simulink model "Model_4"  (R2021b)
settings: Solver=VariableStepAuto  StartTime=0.0  StopTime=10.0  RelTol=1e-3
InitFcn:
  | x_ref = 1; l_ref =0.2; l_ini = 0.7;
  | 
  | %ADRC' s parameter caculation
  | b0 = (ml+mc)/(mc*ml +mc*mt+ml*mt);k_ESO = 15;T_set  = 3;
  | 
  | s_cl = -5.85/T_set;
  | Kp   = s_cl^2;
  | Kd   = -2*s_cl;
  | 
  | s_ESO = k_ESO*s_cl;
  | l1        = -3*s_ESO;
  | l2        = 3*( s_ESO)^2;
  | l3        = -(s_ESO)^3;
  | 
  | %Observer
  | A = [-l1, 1, 0;
  |         -l2, 0, 1;
  |         -l3, 0, 0];
  | B = [0;
  |         b0;
  |         0];
  | L = [l1;
  |        l2;
  |        l3];
  | 
  | b1 = (mt+mc)/(mc*ml +mc*mt+ml*mt);k_ESO1 =90;T_set1  =3;
  | s_cl1 = -5.85/T_set1;
  | Kp1   = s_cl1^2;
  | Kd1   = -2*s_cl1;
  | 
  | s_ESO1 = k_ESO1*s_cl1;
  | l11        = -3*s_ESO1;
  | l21        = 3*( s_ESO1)^2;
  | l31        = -(s_ESO1)^3;
  | 
  | %Observer
  | A1 = [-l11, 1, 0;
  |         -l21, 0, 1;
  |         -l31, 0, 0];
  | B1 = [0;
  |         b1;
  |         0];
  | L1 = [l11;
  |        l21;
  |        l31];
values from neighbouring files (symbols this model uses):
  g = 9.81    [Thong_so_double_pendulum.m]
undefined symbols (not defined in the file or in its folder): data_model41, i, l, mc, o, particle, sigbuilder_block
libraries: neural x166, simulink x5, simulink_extras x5
(part 1 of 4)
settings Model: Creator=Dao Hieu  LastModifiedBy=Admin

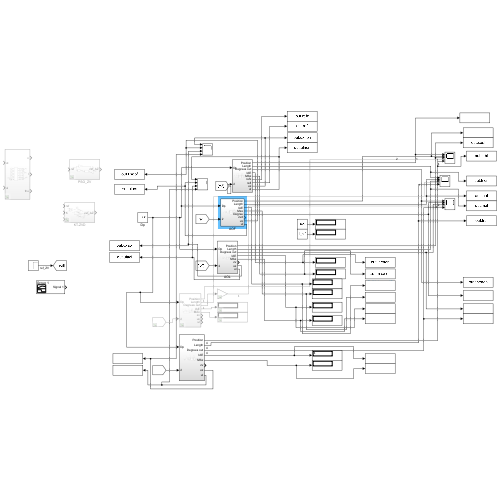
[thumbnail: Simulink's stored preview of the top-level diagram]
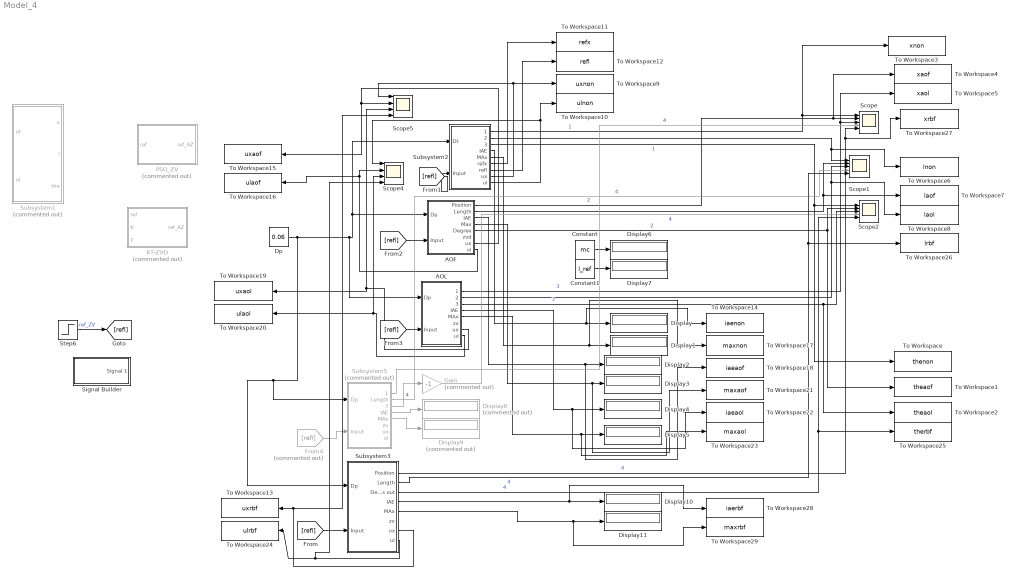
== system Model_4 ==
  AOF : Subsystem
  AOL : Subsystem
  Constant : Constant  Value=mc
  Constant1 : Constant  Value=l_ref
  Display{,1..7,10..11} (10 alike) : Display
  Display8 : Display  Commented=on
  Display9 : Display  Commented=on
  Dp : Constant  Value=0.06
  From4 : From  Commented=on  GotoTag=refl
  Gain : Gain  Commented=on  Gain=-1
  KT-ZVD : Subsystem  Commented=on
  PSO_ZV : Subsystem  Commented=on
  Scope : Scope  NumInputPorts=5
  Scope1 : Scope  NumInputPorts=5
  Scope2 : Scope  NumInputPorts=5
  Scope4 : Scope  NumInputPorts=4
  Scope5 : Scope  NumInputPorts=4
  Signal Builder : Subsystem  Tag=STV Subsys  LoadFcn=sigbuilder_block('load');  StartFcn=sigbuilder_block('start');  StopFcn=sigbuilder_block('stop');  ClipboardFcn=sigbuilder_block('clipboard');  mask(Sigbuilder block){tuvar=[0:10]}
      mask help: Simulink:masks:SigbuilderBlock_MD
      mask init:
      | if ~strcmp(get_param(bdroot(gcbh),'SimulationStatus'),'stopped') tuvar = sigbuilder_block('maskInit'); end
      settings: CopyFcn=sigbuilder_block('copy');  DeleteFcn=sigbuilder_block('delete');  ModelCloseFcn=sigbuilder_block('modelClose');  PreSaveFcn=sigbuilder_block('preSave');  PauseFcn=sigbuilder_block('pause');  ContinueFcn=sigbuilder_block('continue');  NameChangeFcn=sigbuilder_block('namechange');  OpenFcn=sigbuilder_block('open',[388.2 157.8 550.8 400.2 ]);  CloseFcn=sigbuilder_block('close');
      mask Display: plot(0, 0, 100, 100,[2, 2, 32, 32, 2], [68, 8, 8, 68, 68],[32, 2], [38, 38], [32, 19, 2],[53, 60, 44], [32, 17, 17, 2],[16, 16, 31, 31]);txt = getActiveGroup(gcbh);text(2, 100, txt,'verticalAlignment', 'top');
  Step6 : Step  Before=l_ini  After=l_ref  SampleTime=0
  Subsystem1 : Subsystem  Commented=on
  Subsystem2 : Subsystem
  Subsystem3 : Subsystem
  Subsystem5 : Subsystem  Commented=on
  To Workspace : ToWorkspace  VariableName=thenon  SampleTime=0.001
  To Workspace1 : ToWorkspace  VariableName=theaof  SampleTime=0.001
  To Workspace10 : ToWorkspace  VariableName=ulnon  SampleTime=0.001
  To Workspace11 : ToWorkspace  VariableName=refx  SampleTime=0.001
  To Workspace12 : ToWorkspace  VariableName=refl  SampleTime=0.001
  To Workspace13 : ToWorkspace  VariableName=uxrbf  SampleTime=0.001
  To Workspace14 : ToWorkspace  VariableName=iaenon  SampleTime=0.1
  To Workspace15 : ToWorkspace  VariableName=uxaof  SampleTime=0.001
  To Workspace16 : ToWorkspace  VariableName=ulaof  SampleTime=0.001
  To Workspace17 : ToWorkspace  VariableName=maxnon  SampleTime=0.1
  To Workspace18 : ToWorkspace  VariableName=iaeaof  SampleTime=0.1
  To Workspace19 : ToWorkspace  VariableName=uxaol  SampleTime=0.001
  To Workspace2 : ToWorkspace  VariableName=theaol  SampleTime=0.001
  To Workspace20 : ToWorkspace  VariableName=ulaol  SampleTime=0.001
  To Workspace21 : ToWorkspace  VariableName=maxaof  SampleTime=0.1
  To Workspace22 : ToWorkspace  VariableName=iaeaol  SampleTime=0.1
  To Workspace23 : ToWorkspace  VariableName=maxaol  SampleTime=0.1
  To Workspace24 : ToWorkspace  VariableName=ulrbf  SampleTime=0.001
  To Workspace25 : ToWorkspace  VariableName=therbf  SampleTime=0.001
  To Workspace26 : ToWorkspace  VariableName=lrbf  SampleTime=0.001
  To Workspace27 : ToWorkspace  VariableName=xrbf  SampleTime=0.001
  To Workspace28 : ToWorkspace  VariableName=iaerbf  SampleTime=0.1
  To Workspace29 : ToWorkspace  VariableName=maxrbf  SampleTime=0.1
  To Workspace3 : ToWorkspace  VariableName=xnon  SampleTime=0.001
  To Workspace4 : ToWorkspace  VariableName=xaof  SampleTime=0.001
  To Workspace5 : ToWorkspace  VariableName=xaol  SampleTime=0.001
  To Workspace6 : ToWorkspace  VariableName=lnon  SampleTime=0.001
  To Workspace7 : ToWorkspace  VariableName=laof  SampleTime=0.001
  To Workspace8 : ToWorkspace  VariableName=laol  SampleTime=0.001
  To Workspace9 : ToWorkspace  VariableName=uxnon  SampleTime=0.001
  wires:
  AOF/3(IAE) -> To Workspace18/1, Display2/1
  AOF/4(Max) -> To Workspace21/1, Display3/1
  Subsystem2/1(Position) -> To Workspace3/1, Scope/1  "1"
  Subsystem2/2(Length) -> To Workspace6/1, Scope1/1
  Subsystem2/3(Degrees out) -> To Workspace/1, Scope2/1  "1"
  Subsystem2/4(IAE) -> To Workspace14/1, Display/1
  Subsystem2/5(MAx) -> To Workspace17/1, Display1/1
  AOL/4(IAE) -> To Workspace22/1, Display4/1
  AOF/1(Position) -> To Workspace4/1, Scope/2  "2"
  AOL/1(Position) -> To Workspace5/1, Scope/3  "3"
  AOF/2(Length) -> Scope1/2, To Workspace7/1
  AOL/2(Length) -> To Workspace8/1, Scope1/3
  AOL/3(Degrees out) -> To Workspace2/1, Scope2/3  "3"
  AOF/5(Degree) -> Scope2/2, To Workspace1/1  "2"
  Subsystem2/6(refx) -> To Workspace11/1
  Subsystem2/7(refl) -> To Workspace12/1
  Subsystem2/8(ux) -> Scope5/1, To Workspace9/1
  Subsystem2/9(ul) -> To Workspace10/1, Scope4/1
  AOF/7(ux) -> Scope5/2, To Workspace15/1
  AOF/8(ul) -> Scope4/2, To Workspace16/1
  AOL/7(ux) -> Scope5/3, To Workspace19/1
  AOL/8(ul) -> Scope4/3, To Workspace20/1
  AOL/5(MAx) -> To Workspace23/1, Display5/1
  Constant/1 -> Display6/1
  Constant1/1 -> Display7/1
  Dp/1 -> AOL/1(Dp), AOF/1(Dp), Subsystem2/1(Dt), Subsystem5/1(Dp), Subsystem3/1(Dp)
  Subsystem5/1(Position) -> Scope/4  "4"
  Subsystem5/2(Length) -> Scope1/4  "4"
  Subsystem5/3(Degrees out) -> Gain/1  "4"
  Gain/1 -> Scope2/4  "4"
  Subsystem3/3(Degrees out) -> To Workspace25/1, Scope2/5  "4"
  Subsystem3/1(Position) -> To Workspace27/1, Scope/5  "4"
  Subsystem3/2(Length) -> To Workspace26/1, Scope1/5  "4"
  Subsystem5/4(IAE) -> Display8/1
  Subsystem5/5(MAx) -> Display9/1
  Subsystem3/4(IAE) -> To Workspace28/1, Display10/1
  Subsystem3/5(MAx) -> To Workspace29/1, Display11/1
  Step6/1 -> [refl]  "ref_ZV"
  [refl] -> Subsystem2/2(Input)
  [refl] -> AOF/2(Input)
  [refl] -> AOL/2(Input)
  From4/1 -> Subsystem5/2(Input)
  [refl] -> Subsystem3/2(Input)
  Subsystem3/7(ux) -> Scope5/4, To Workspace13/1
  Subsystem3/8(ul) -> Scope4/4, To Workspace24/1

== system Model_4/AOF ==
  Dp : Inport
  Input : Inport  Port=2
  ADRC 1 : Subsystem
  ADRC 2 : Subsystem
  Constant3 : Constant  Value=pi/(0.5*(sqrt(9.81/l_ini)+sqrt(9.81/l_ref)))
  Constant4 : Constant  Value=2*pi/(0.5*(sqrt(9.81/l_ini)+sqrt(9.81/l_ref)))
  Fitness APS ZVD1 : Subsystem
  Gain2 : Gain  Gain=-0.5
  Radians to Degrees1 : simulink_extras/Transformations/Radians to Degrees
  Saturation : Saturate  UpperLimit=inf  LowerLimit=0
  Step1 : Step  After=x_ref  SampleTime=0
  Subsystem2 : Subsystem
  ZVD1 : Subsystem
  Position : Outport
  Length : Outport  Port=2
  IAE : Outport  Port=3
  Max : Outport  Port=4
  Degree : Outport  Port=5
  zvd : Outport  Port=6
  ux : Outport  Port=7
  ul : Outport  Port=8
  wires:
  Subsystem2/1(x) -> ADRC 2/2(x), Position/1  "Position"
  Dp/1 -> Subsystem2/3(Dt)
  ADRC 1/1(u) -> ul/1, Subsystem2/2(ul)  "ADRC"
  ADRC 2/1(u) -> ux/1, Subsystem2/1(ut)  "ADRC"
  Input/1 -> ADRC 1/1(ref)  "ref_ZV"
  Step1/1 -> ZVD1/1(ref)  "ref_ZV"
  ZVD1/1(ref_AZ) -> zvd/1, ADRC 2/1(ref)  "ref_ZV"
  Subsystem2/3(the) -> Gain2/1
  Constant4/1 -> ZVD1/3(Input1)
  Constant3/1 -> ZVD1/2(Input)
  Radians to Degrees1/1 -> Degree/1, Fitness APS ZVD1/1(e)
  Fitness APS ZVD1/2(MAx) -> Max/1
  Fitness APS ZVD1/1(IAE) -> IAE/1
  Gain2/1 -> Radians to Degrees1/1
  Subsystem2/2(l) -> Saturation/1  "Length"
  Saturation/1 -> ADRC 1/2(x), Length/1

== system Model_4/AOL ==
  Dp : Inport
  Input : Inport  Port=2
  "ADRC " : Subsystem
  ADRC 1 : Subsystem
  Constant : Constant  Value=pi/sqrt(9.81/((l_ini+l_ref)/2))
  Constant1 : Constant  Commented=on  Value=data_model41(int8((l_ref-0.2)/0.01+1),2)
  Constant2 : Constant  Commented=on  Value=data_model41(int8((l_ref-0.2)/0.01+1),3)
  Constant3 : Constant  Commented=on  Value=data_model41(o,1)
  Constant4 : Constant  Commented=on  Value=data_model41(o,2)
  Constant5 : Constant  Value=2*pi/sqrt(9.81/((l_ini+l_ref)/2))
  Fitness APS ZVD : Subsystem
  Gain : Gain  Gain=-0.5
  Radians to Degrees : simulink_extras/Transformations/Radians to Degrees
  Saturation : Saturate  UpperLimit=inf  LowerLimit=0
  Step5 : Step  After=x_ref  SampleTime=0
  Subsystem : Subsystem
  ZVD1 : Subsystem
  ZVD3 : Subsystem  Commented=on
  Position : Outport
  Length : Outport  Port=2
  Degrees out : Outport  Port=3
  IAE : Outport  Port=4
  MAx : Outport  Port=5
  zv : Outport  Port=6
  ux : Outport  Port=7
  ul : Outport  Port=8
  wires:
  Subsystem/3(the) -> Radians to Degrees/1
  Radians to Degrees/1 -> Gain/1
  Fitness APS ZVD/1(IAE) -> IAE/1
  Dp/1 -> Subsystem/3(Dt)
  Subsystem/1(x) -> Position/1, "ADRC "/2(x)  "Position"
  "ADRC "/1(u) -> ux/1, Subsystem/1(ut)  "ADRC"
  ADRC 1/1(u) -> ul/1, Subsystem/2(ul)  "ADRC"
  Input/1 -> ADRC 1/1(ref)  "ref_ZV"
  Step5/1 -> ZVD1/1(ref)  "ref_ZV"
  ZVD1/1(ref_AZ) -> zv/1, "ADRC "/1(ref)  "ref_ZV"
  Fitness APS ZVD/2(MAx) -> MAx/1
  Gain/1 -> Degrees out/1, Fitness APS ZVD/1(e)
  Constant/1 -> ZVD1/2(Input)
  Constant5/1 -> ZVD1/3(Input1)
  Subsystem/2(l) -> Saturation/1  "Length"
  Saturation/1 -> ADRC 1/2(x), Length/1

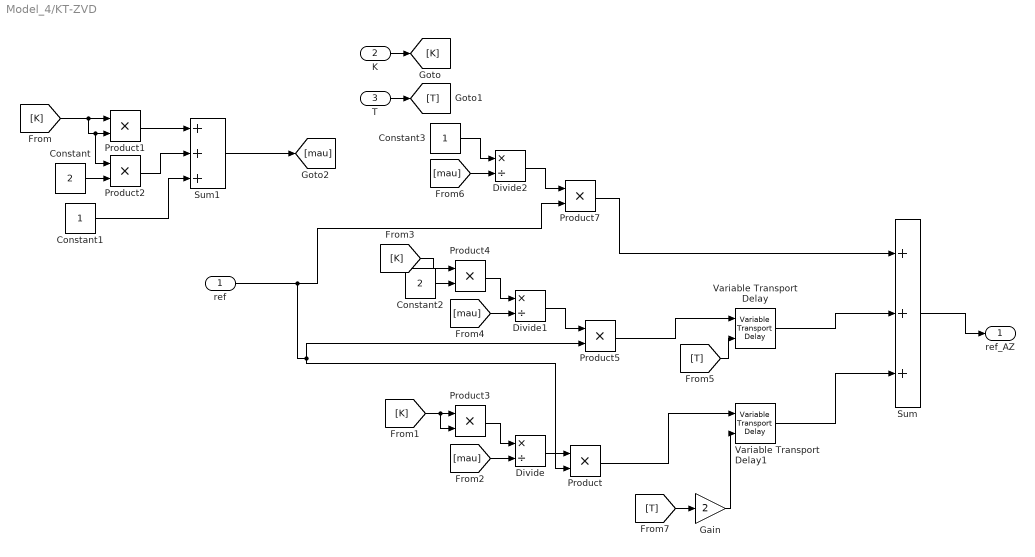
== system Model_4/KT-ZVD ==
  ref : Inport
  K : Inport  Port=2
  T : Inport  Port=3
  Constant : Constant  Value=2
  Constant1 : Constant
  Constant2 : Constant  Value=2
  Constant3 : Constant
  Divide : Product  Inputs=*/
  Divide1 : Product  Inputs=*/
  Divide2 : Product  Inputs=*/
  Gain : Gain  Gain=2
  Product{,1..5,7} (7 alike) : Product
  Sum : Sum  Inputs=+++
  Sum1 : Sum  Inputs=+++
  Variable Transport Delay : VariableTransportDelay  VariableDelayType=Variable transport delay  MaximumDelay=10
  Variable Transport Delay1 : VariableTransportDelay  VariableDelayType=Variable transport delay  MaximumDelay=10
  ref_AZ : Outport
  wires:
  Product5/1 -> Variable Transport Delay/1
  Product7/1 -> Sum/1
  Variable Transport Delay/1 -> Sum/2
  Sum/1 -> ref_AZ/1
  ref/1 -> Product7/2, Product/2, Product5/2
  Product/1 -> Variable Transport Delay1/1
  Variable Transport Delay1/1 -> Sum/3
  K/1 -> [K]
  T/1 -> [T]
  [K] -> Product2/1, Product1/2, Product1/1
  Constant/1 -> Product2/2
  Product1/1 -> Sum1/1
  Product2/1 -> Sum1/2
  Constant1/1 -> Sum1/3
  Sum1/1 -> [mau]
  [K] -> Product4/1
  Product4/1 -> Divide1/1
  [mau] -> Divide1/2
  Divide1/1 -> Product5/1
  Constant2/1 -> Product4/2
  Constant3/1 -> Divide2/1
  Divide2/1 -> Product7/1
  [mau] -> Divide2/2
  [K] -> Product3/2, Product3/1
  Product3/1 -> Divide/1
  [mau] -> Divide/2
  Divide/1 -> Product/1
  [T] -> Variable Transport Delay/2
  [T] -> Gain/1
  Gain/1 -> Variable Transport Delay1/2

== system Model_4/PSO_ZV ==
  ref : Inport
  Gain : Gain  Gain=1/((particle(i).Position(1,1))+1)
  Gain1 : Gain  Gain=(particle(i).Position(1,1))/((particle(i).Position(1,1))+1)
  Sum : Sum
  Transport Delay : TransportDelay  DelayTime=particle(i).Position(1,2)
  ref_AZ : Outport
  wires:
  Gain1/1 -> Transport Delay/1
  Gain/1 -> Sum/1
  Transport Delay/1 -> Sum/2
  Sum/1 -> ref_AZ/1
  ref/1 -> Gain/1, Gain1/1

== system Model_4/Signal Builder ==
  Demux : Demux  Tag=STV Demux  Outputs=1
      settings: DisplayOption=none
  FromWs : FromWorkspace  Tag=STV FromWs  VariableName=tuvar
      SigBuilderData=|
      | common.afterFinalStr = 'Extrapolate'
      | common.sampleTime = 0
      | dataSet.timeRange = [0 10]
      | dataSet.name = 'Group 1'
      | sbobj.Groups.Name = 'Group 1'
      | sbobj.Groups.Signals.Name = 'Signal 1'
      | sbobj.Groups.Signals.XData = [0 1 1 3 3 10]
      | sbobj.Groups.Signals.YData = [0.7 0.7 0.2 0.2 0.7 0.7]
  Signal 1 : Outport  Tag=STV Outport
  wires:
  Demux/1 -> Signal 1/1
  FromWs/1 -> Demux/1

== system Model_4/Subsystem1 ==
  ut : Inport
  ul : Inport  Port=2
  Add : Sum
  Constant : Constant  Value=-mc*g
  Crane : MATLAB Function  TreatAsAtomicUnit=on
  Integrator{,1,3..5} (5 alike) : Integrator
  Integrator2 : Integrator  InitialCondition=l
  x : Outport
  l : Outport  Port=2
  the : Outport  Port=3
  wires:
  Integrator5/1 -> [x6]
  Integrator2/1 -> l/1, [x3]
  [x4] -> Crane/4(x4)
  Crane/5(dx5) -> Integrator4/1
  Crane/6(dx6) -> Integrator5/1
  Crane/1(dx1) -> Integrator/1
  Crane/3(dx3) -> Integrator2/1
  Integrator1/1 -> [x2]
  [x2] -> Crane/2(x2)
  Integrator4/1 -> the/1, [x5]
  [x3] -> Crane/3(x3)
  [x6] -> Crane/6(x6)
  [x5] -> Crane/5(x5)
  Crane/4(dx4) -> Integrator3/1
  Integrator/1 -> x/1, [x1]
  Integrator3/1 -> [x4]
  [x1] -> Crane/1(x1)
  Crane/2(dx2) -> Integrator1/1
  ut/1 -> Crane/7(ut)
  ul/1 -> Add/2
  Constant/1 -> Add/1
  Add/1 -> Crane/8(ul)

== system Model_4/Subsystem2 ==
  Dt : Inport
  Input : Inport  Port=2
  "ADRC " : Subsystem
  ADRC 1 : Subsystem
  Fitness APS ZVD : Subsystem
  Gain2 : Gain  Gain=-0.5
  Radians to Degrees : simulink_extras/Transformations/Radians to Degrees
  Saturation : Saturate  UpperLimit=inf  LowerLimit=0
  Step5 : Step  After=x_ref  SampleTime=0
  Subsystem : Subsystem
  Position : Outport
  Length : Outport  Port=2
  Degrees out : Outport  Port=3
  IAE : Outport  Port=4
  MAx : Outport  Port=5
  refx : Outport  Port=6
  refl : Outport  Port=7
  ux : Outport  Port=8
  ul : Outport  Port=9
  wires:
  Radians to Degrees/1 -> Degrees out/1, Fitness APS ZVD/1(e)
  Fitness APS ZVD/1(IAE) -> IAE/1
  Dt/1 -> Subsystem/3(Dt)
  Subsystem/1(x) -> Position/1, "ADRC "/2(x)  "Position"
  "ADRC "/1(u) -> ux/1, Subsystem/1(ut)  "ADRC"
  ADRC 1/1(u) -> ul/1, Subsystem/2(ul)  "ADRC"
  Input/1 -> refl/1, ADRC 1/1(ref)  "ref_ZV"
  Step5/1 -> refx/1, "ADRC "/1(ref)  "ref_ZV"
  Fitness APS ZVD/2(MAx) -> MAx/1
  Subsystem/3(the) -> Gain2/1
  Gain2/1 -> Radians to Degrees/1
  Subsystem/2(l) -> Saturation/1  "Length"
  Saturation/1 -> ADRC 1/2(x), Length/1

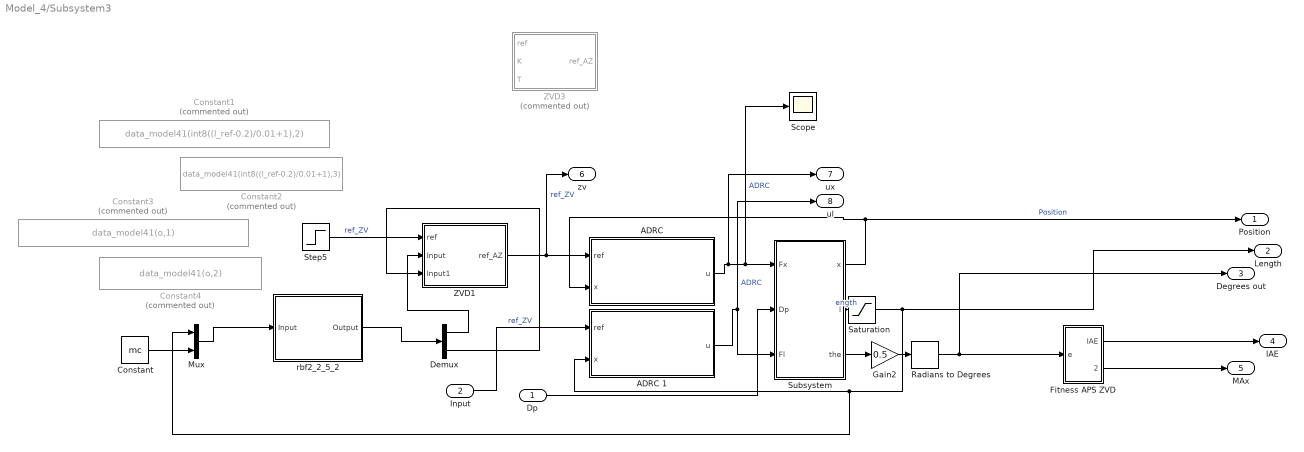
== system Model_4/Subsystem3 ==
  Dp : Inport
  Input : Inport  Port=2
  "ADRC " : Subsystem
  ADRC 1 : Subsystem
  Constant : Constant  Value=mc
  Constant1 : Constant  Commented=on  Value=data_model41(int8((l_ref-0.2)/0.01+1),2)
  Constant2 : Constant  Commented=on  Value=data_model41(int8((l_ref-0.2)/0.01+1),3)
  Constant3 : Constant  Commented=on  Value=data_model41(o,1)
  Constant4 : Constant  Commented=on  Value=data_model41(o,2)
  Demux : Demux  Outputs=2
  Fitness APS ZVD : Subsystem
  Gain2 : Gain  Gain=0.5
  Mux : Mux  Inputs=2
  Radians to Degrees : simulink_extras/Transformations/Radians to Degrees
  Saturation : Saturate  UpperLimit=inf  LowerLimit=0
  Scope : Scope
  Step5 : Step  After=x_ref  SampleTime=0
  Subsystem : Subsystem
  ZVD1 : Subsystem
  ZVD3 : Subsystem  Commented=on
  rbf2_2_5_2 : Subsystem
      mask help: Radial Basis Network
      mask Display: e = 0.06;c1 = [120 150 230]/255;c2 = ([120 150 230]+0)/383;c3 = ([120 150 230]+128)/383;patch([0 1 1 0],[0 0 1 1],c1);patch([0 1 1 1-e 1-e 0+e],[0 0 1 1-e 0+e 0+e],c2);patch([0 0 1 1-e 0+e 0+e],[0 1 1 1-e 1-e 0+e],c3);plot([0 1 1 0 0],[0 0 1 1 0]);fprintf('NNET');port_label('input',1,' Input');port_label('output',1,'Output ');
  Position : Outport
  Length : Outport  Port=2
  Degrees out : Outport  Port=3
  IAE : Outport  Port=4
  MAx : Outport  Port=5
  zv : Outport  Port=6
  ux : Outport  Port=7
  ul : Outport  Port=8
  wires:
  Fitness APS ZVD/1(IAE) -> IAE/1
  Dp/1 -> Subsystem/2(Dp)
  Subsystem/1(x) -> "ADRC "/2(x), Position/1  "Position"
  "ADRC "/1(u) -> ux/1, Scope/1, Subsystem/1(Fx)  "ADRC"
  ADRC 1/1(u) -> Subsystem/3(Fl), ul/1  "ADRC"
  Input/1 -> ADRC 1/1(ref)  "ref_ZV"
  Step5/1 -> ZVD1/1(ref)  "ref_ZV"
  ZVD1/1(ref_AZ) -> zv/1, "ADRC "/1(ref)  "ref_ZV"
  Fitness APS ZVD/2(MAx) -> MAx/1
  Radians to Degrees/1 -> Degrees out/1, Fitness APS ZVD/1(e)
  rbf2_2_5_2/1(Output) -> Demux/1
  Demux/1 -> ZVD1/2(Input)
  Demux/2 -> ZVD1/3(Input1)
  Mux/1 -> rbf2_2_5_2/1(Input)
  Constant/1 -> Mux/2
  Subsystem/3(the) -> Gain2/1
  Gain2/1 -> Radians to Degrees/1
  Subsystem/2(l) -> Saturation/1  "ength"
  Saturation/1 -> Mux/1, ADRC 1/2(x), Length/1

== system Model_4/Subsystem5 ==
  Dp : Inport
  Input : Inport  Port=2
  "ADRC " : Subsystem
  ADRC 1 : Subsystem
  Constant : Constant  Value=mc
  Constant1 : Constant  Commented=on  Value=data_model41(int8((l_ref-0.2)/0.01+1),2)
  Constant2 : Constant  Commented=on  Value=data_model41(int8((l_ref-0.2)/0.01+1),3)
  Constant3 : Constant  Commented=on  Value=data_model41(o,1)
  Constant4 : Constant  Commented=on  Value=data_model41(o,2)
  Demux : Demux  Outputs=2
  Fitness APS ZVD : Subsystem
  Gain2 : Gain  Gain=0.5
  Mux : Mux  Inputs=2
  Radial Basis Network : Subsystem
      mask help: Radial Basis Network
      mask Display: e = 0.06;c1 = [120 150 230]/255;c2 = ([120 150 230]+0)/383;c3 = ([120 150 230]+128)/383;patch([0 1 1 0],[0 0 1 1],c1);patch([0 1 1 1-e 1-e 0+e],[0 0 1 1-e 0+e 0+e],c2);patch([0 0 1 1-e 0+e 0+e],[0 1 1 1-e 1-e 0+e],c3);plot([0 1 1 0 0],[0 0 1 1 0]);fprintf('NNET');port_label('input',1,' Input');port_label('output',1,'Output ');
  Radians to Degrees : simulink_extras/Transformations/Radians to Degrees
  Scope : Scope
  Step5 : Step  After=x_ref  SampleTime=0
  Subsystem : Subsystem
  ZVD1 : Subsystem
  ZVD3 : Subsystem  Commented=on
  Position : Outport
  Length : Outport  Port=2
  Degrees out : Outport  Port=3
  IAE : Outport  Port=4
  MAx : Outport  Port=5
  zv : Outport  Port=6
  ux : Outport  Port=7
  ul : Outport  Port=8
  wires:
  Fitness APS ZVD/1(IAE) -> IAE/1
  Dp/1 -> Subsystem/3(Dp)
  Subsystem/1(x) -> Position/1, "ADRC "/2(x)  "Position"
  Subsystem/2(l) -> Mux/1, ADRC 1/2(x), Length/1  "Length"
  "ADRC "/1(u) -> ux/1, Scope/1, Subsystem/1(Fx)  "ADRC"
  ADRC 1/1(u) -> ul/1, Subsystem/2(Fl)  "ADRC"
  Input/1 -> ADRC 1/1(ref)  "ref_ZV"
  Step5/1 -> ZVD1/1(ref)  "ref_ZV"
  ZVD1/1(ref_AZ) -> zv/1, "ADRC "/1(ref)  "ref_ZV"
  Fitness APS ZVD/2(MAx) -> MAx/1
  Radians to Degrees/1 -> Degrees out/1, Fitness APS ZVD/1(e)
  Radial Basis Network/1(Output) -> Demux/1
  Demux/1 -> ZVD1/2(Input)
  Demux/2 -> ZVD1/3(Input1)
  Mux/1 -> Radial Basis Network/1(Input)
  Constant/1 -> Mux/2
  Subsystem/3(the) -> Gain2/1
  Gain2/1 -> Radians to Degrees/1

== system Model_4/AOF/ADRC 1 ==
  ref : Inport
  x : Inport  Port=2
  Gain : Gain  Gain=Kp1
  Gain1 : Gain  Gain=Kd1
  Gain2 : Gain  Gain=1/b1
  Observer : Subsystem
  Sum : Sum  Inputs=|+-
  Sum3 : Sum  Inputs=|+-
  Sum4 : Sum  Inputs=|+-
  u : Outport
  wires:
  Sum4/1 -> Gain2/1
  Sum/1 -> Gain/1
  Gain2/1 -> u/1, Observer/1(u)
  x/1 -> Observer/2(x)
  Sum3/1 -> Sum4/1
  Observer/2(x2) -> Gain1/1
  Gain1/1 -> Sum3/2
  Gain/1 -> Sum3/1
  ref/1 -> Sum/1
  Observer/1(x3) -> Sum4/2
  Observer/3(x1) -> Sum/2

== system Model_4/AOF/ADRC 2 ==
  ref : Inport
  x : Inport  Port=2
  Gain : Gain  Gain=Kp
  Gain1 : Gain  Gain=Kd
  Gain2 : Gain  Gain=1/b0
  Observer : Subsystem
  Sum : Sum  Inputs=|+-
  Sum3 : Sum  Inputs=|+-
  Sum4 : Sum  Inputs=|+-
  u : Outport
  wires:
  Sum4/1 -> Gain2/1
  Sum/1 -> Gain/1
  Gain2/1 -> u/1, Observer/1(u)
  x/1 -> Observer/2(x)
  Sum3/1 -> Sum4/1
  Observer/2(x2) -> Gain1/1
  Gain1/1 -> Sum3/2
  Gain/1 -> Sum3/1
  ref/1 -> Sum/1
  Observer/1(x3) -> Sum4/2
  Observer/3(x1) -> Sum/2

== system Model_4/AOF/Fitness APS ZVD1 ==
  e : Inport
  Abs : Abs
  Abs1 : Abs
  Integrator : Integrator
  MinMax Running Resettable : simulink/Math Operations/MinMax Running Resettable  Function=max  vinit=0.0
  Step : Step  Time=0.000001  Before=1  After=0  SampleTime=0
  IAE : Outport
  MAx : Outport  Port=2
  wires:
  Abs/1 -> Integrator/1
  Abs1/1 -> MinMax Running Resettable/1
  Step/1 -> MinMax Running Resettable/2
  e/1 -> Abs/1, Abs1/1
  Integrator/1 -> IAE/1
  MinMax Running Resettable/1 -> MAx/1

== system Model_4/AOF/Subsystem2 ==
  ut : Inport
  ul : Inport  Port=2
  Dt : Inport  Port=3
  Add : Sum
  Constant : Constant  Value=-mc*g
  Constant1 : Constant  Value=mc
  Crane : MATLAB Function  TreatAsAtomicUnit=on
  Integrator{,1,3..5} (5 alike) : Integrator
  Integrator2 : Integrator  InitialCondition=l_ini
  x : Outport
  l : Outport  Port=2
  the : Outport  Port=3
  wires:
  Integrator5/1 -> [x6]
  Integrator2/1 -> l/1, [x3]
  [x4] -> Crane/3(x4)
  Crane/5(dx5) -> Integrator4/1
  Crane/6(dx6) -> Integrator5/1
  Crane/1(dx1) -> Integrator/1
  Crane/3(dx3) -> Integrator2/1
  Integrator1/1 -> [x2]
  [x2] -> Crane/1(x2)
  Integrator4/1 -> the/1, [x5]
  [x3] -> Crane/2(x3)
  [x6] -> Crane/5(x6)
  [x5] -> Crane/4(x5)
  Crane/4(dx4) -> Integrator3/1
  Integrator/1 -> x/1, [x1]
  Integrator3/1 -> [x4]
  Crane/2(dx2) -> Integrator1/1
  ut/1 -> Crane/6(ut)
  ul/1 -> Add/2
  Constant/1 -> Add/1
  Add/1 -> Crane/7(ul)
  Dt/1 -> Crane/8(Dt)
  Constant1/1 -> Crane/9(mc)

== system Model_4/AOF/ZVD1 ==
  ref : Inport
  Input : Inport  Port=2
  Input1 : Inport  Port=3
  Gain1 : Gain  Gain=0.25
  Gain2 : Gain  Gain=0.5
  Gain3 : Gain  Gain=0.25
  MATLAB Function : MATLAB Function  Commented=on  TreatAsAtomicUnit=on
  MATLAB Function1 : MATLAB Function  Commented=on  TreatAsAtomicUnit=on
  Sum : Sum  Inputs=+++
  Variable Transport Delay : VariableTransportDelay  VariableDelayType=Variable transport delay  MaximumDelay=10
  Variable Transport Delay1 : VariableTransportDelay  VariableDelayType=Variable transport delay  MaximumDelay=10
  ref_AZ : Outport
  wires:
  Gain2/1 -> Variable Transport Delay/1
  Gain1/1 -> Sum/1
  Variable Transport Delay/1 -> Sum/2
  Sum/1 -> ref_AZ/1
  ref/1 -> Gain1/1, Gain3/1, Gain2/1
  Gain3/1 -> Variable Transport Delay1/1
  Variable Transport Delay1/1 -> Sum/3
  Input/1 -> Variable Transport Delay/2
  MATLAB Function1/1(y) -> ?
  Input1/1 -> Variable Transport Delay1/2

== system Model_4/AOL/ADRC  ==
  ref : Inport
  x : Inport  Port=2
  Gain : Gain  Gain=Kp
  Gain1 : Gain  Gain=Kd
  Gain2 : Gain  Gain=1/b0
  Observer : Subsystem
  Sum : Sum  Inputs=|+-
  Sum3 : Sum  Inputs=|+-
  Sum4 : Sum  Inputs=|+-
  u : Outport
  wires:
  Sum4/1 -> Gain2/1
  Sum/1 -> Gain/1
  Gain2/1 -> u/1, Observer/1(u)
  x/1 -> Observer/2(x)
  Sum3/1 -> Sum4/1
  Observer/2(x2) -> Gain1/1
  Gain1/1 -> Sum3/2
  Gain/1 -> Sum3/1
  ref/1 -> Sum/1
  Observer/1(x3) -> Sum4/2
  Observer/3(x1) -> Sum/2

== system Model_4/AOL/ADRC 1 ==
  ref : Inport
  x : Inport  Port=2
  Gain : Gain  Gain=Kp1
  Gain1 : Gain  Gain=Kd1
  Gain2 : Gain  Gain=1/b1
  Observer : Subsystem
  Sum : Sum  Inputs=|+-
  Sum3 : Sum  Inputs=|+-
  Sum4 : Sum  Inputs=|+-
  u : Outport
  wires:
  Sum4/1 -> Gain2/1
  Sum/1 -> Gain/1
  Gain2/1 -> u/1, Observer/1(u)
  x/1 -> Observer/2(x)
  Sum3/1 -> Sum4/1
  Observer/2(x2) -> Gain1/1
  Gain1/1 -> Sum3/2
  Gain/1 -> Sum3/1
  ref/1 -> Sum/1
  Observer/1(x3) -> Sum4/2
  Observer/3(x1) -> Sum/2

== system Model_4/AOL/Fitness APS ZVD ==
  e : Inport
  Abs : Abs
  Abs1 : Abs
  Integrator : Integrator
  MinMax Running Resettable : simulink/Math Operations/MinMax Running Resettable  Function=max  vinit=0.0
  Step : Step  Time=0.000001  Before=1  After=0  SampleTime=0
  IAE : Outport
  MAx : Outport  Port=2
  wires:
  Abs/1 -> Integrator/1
  Abs1/1 -> MinMax Running Resettable/1
  Step/1 -> MinMax Running Resettable/2
  e/1 -> Abs/1, Abs1/1
  Integrator/1 -> IAE/1
  MinMax Running Resettable/1 -> MAx/1

== system Model_4/AOL/Subsystem ==
  ut : Inport
  ul : Inport  Port=2
  Dt : Inport  Port=3
  Add : Sum
  Constant : Constant  Value=-mc*g
  Constant1 : Constant  Value=mc
  Crane : MATLAB Function  TreatAsAtomicUnit=on
  Integrator{,1,3..5} (5 alike) : Integrator
  Integrator2 : Integrator  InitialCondition=l_ini
  x : Outport
  l : Outport  Port=2
  the : Outport  Port=3
  wires:
  Integrator5/1 -> [x6]
  Integrator2/1 -> l/1, [x3]
  [x4] -> Crane/3(x4)
  Crane/5(dx5) -> Integrator4/1
  Crane/6(dx6) -> Integrator5/1
  Crane/1(dx1) -> Integrator/1
  Crane/3(dx3) -> Integrator2/1
  Integrator1/1 -> [x2]
  [x2] -> Crane/1(x2)
  Integrator4/1 -> the/1, [x5]
  [x3] -> Crane/2(x3)
  [x6] -> Crane/5(x6)
  [x5] -> Crane/4(x5)
  Crane/4(dx4) -> Integrator3/1
  Integrator/1 -> x/1, [x1]
  Integrator3/1 -> [x4]
  Crane/2(dx2) -> Integrator1/1
  ut/1 -> Crane/6(ut)
  ul/1 -> Add/2
  Constant/1 -> Add/1
  Add/1 -> Crane/7(ul)
  Dt/1 -> Crane/8(Dt)
  Constant1/1 -> Crane/9(mc)

== system Model_4/AOL/ZVD1 ==
  ref : Inport
  Input : Inport  Port=2
  Input1 : Inport  Port=3
  Gain1 : Gain  Gain=0.25
  Gain2 : Gain  Gain=0.5
  Gain3 : Gain  Gain=0.25
  MATLAB Function : MATLAB Function  Commented=on  TreatAsAtomicUnit=on
  MATLAB Function1 : MATLAB Function  Commented=on  TreatAsAtomicUnit=on
  Sum : Sum  Inputs=+++
  Variable Transport Delay : VariableTransportDelay  VariableDelayType=Variable transport delay  MaximumDelay=10
  Variable Transport Delay1 : VariableTransportDelay  VariableDelayType=Variable transport delay  MaximumDelay=10
  ref_AZ : Outport
  wires:
  Gain2/1 -> Variable Transport Delay/1
  Gain1/1 -> Sum/1
  Variable Transport Delay/1 -> Sum/2
  Sum/1 -> ref_AZ/1
  ref/1 -> Gain1/1, Gain3/1, Gain2/1
  Gain3/1 -> Variable Transport Delay1/1
  Variable Transport Delay1/1 -> Sum/3
  Input/1 -> Variable Transport Delay/2
  MATLAB Function1/1(y) -> ?
  Input1/1 -> Variable Transport Delay1/2

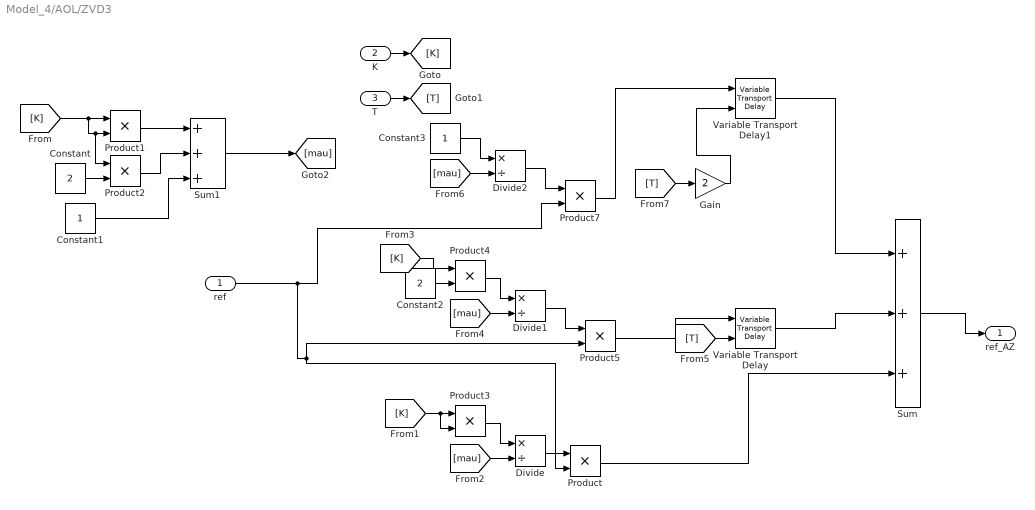
== system Model_4/AOL/ZVD3 ==
  ref : Inport
  K : Inport  Port=2
  T : Inport  Port=3
  Constant : Constant  Value=2
  Constant1 : Constant
  Constant2 : Constant  Value=2
  Constant3 : Constant
  Divide : Product  Inputs=*/
  Divide1 : Product  Inputs=*/
  Divide2 : Product  Inputs=*/
  Gain : Gain  Gain=2
  Product{,1..5,7} (7 alike) : Product
  Sum : Sum  Inputs=+++
  Sum1 : Sum  Inputs=+++
  Variable Transport Delay : VariableTransportDelay  VariableDelayType=Variable transport delay  MaximumDelay=10
  Variable Transport Delay1 : VariableTransportDelay  VariableDelayType=Variable transport delay  MaximumDelay=10
  ref_AZ : Outport
  wires:
  Product5/1 -> Variable Transport Delay/1
  Product7/1 -> Variable Transport Delay1/1
  Variable Transport Delay/1 -> Sum/2
  Sum/1 -> ref_AZ/1
  ref/1 -> Product7/2, Product/2, Product5/2
  Product/1 -> Sum/3
  K/1 -> [K]
  T/1 -> [T]
  [K] -> Product2/1, Product1/2, Product1/1
  Constant/1 -> Product2/2
  Product1/1 -> Sum1/1
  Product2/1 -> Sum1/2
  Constant1/1 -> Sum1/3
  Sum1/1 -> [mau]
  [K] -> Product4/1
  Product4/1 -> Divide1/1
  [mau] -> Divide1/2
  Divide1/1 -> Product5/1
  Constant2/1 -> Product4/2
  Constant3/1 -> Divide2/1
  Divide2/1 -> Product7/1
  [mau] -> Divide2/2
  [K] -> Product3/2, Product3/1
  Product3/1 -> Divide/1
  [mau] -> Divide/2
  Divide/1 -> Product/1
  [T] -> Variable Transport Delay/2
  Gain/1 -> Variable Transport Delay1/2
  [T] -> Gain/1
  Variable Transport Delay1/1 -> Sum/1

== system Model_4/Subsystem2/ADRC  ==
  ref : Inport
  x : Inport  Port=2
  Gain : Gain  Gain=Kp
  Gain1 : Gain  Gain=Kd
  Gain2 : Gain  Gain=1/b0
  Observer : Subsystem
  Sum : Sum  Inputs=|+-
  Sum3 : Sum  Inputs=|+-
  Sum4 : Sum  Inputs=|+-
  u : Outport
  wires:
  Sum4/1 -> Gain2/1
  Sum/1 -> Gain/1
  Gain2/1 -> u/1, Observer/1(u)
  x/1 -> Observer/2(x)
  Sum3/1 -> Sum4/1
  Observer/2(x2) -> Gain1/1
  Gain1/1 -> Sum3/2
  Gain/1 -> Sum3/1
  ref/1 -> Sum/1
  Observer/1(x3) -> Sum4/2
  Observer/3(x1) -> Sum/2

== system Model_4/Subsystem2/ADRC 1 ==
  ref : Inport
  x : Inport  Port=2
  Gain : Gain  Gain=Kp1
  Gain1 : Gain  Gain=Kd1
  Gain2 : Gain  Gain=1/b1
  Observer : Subsystem
  Sum : Sum  Inputs=|+-
  Sum3 : Sum  Inputs=|+-
  Sum4 : Sum  Inputs=|+-
  u : Outport
  wires:
  Sum4/1 -> Gain2/1
  Sum/1 -> Gain/1
  Gain2/1 -> u/1, Observer/1(u)
  x/1 -> Observer/2(x)
  Sum3/1 -> Sum4/1
  Observer/2(x2) -> Gain1/1
  Gain1/1 -> Sum3/2
  Gain/1 -> Sum3/1
  ref/1 -> Sum/1
  Observer/1(x3) -> Sum4/2
  Observer/3(x1) -> Sum/2

== system Model_4/Subsystem2/Fitness APS ZVD ==
  e : Inport
  Abs : Abs
  Abs1 : Abs
  Integrator : Integrator
  MinMax Running Resettable : simulink/Math Operations/MinMax Running Resettable  Function=max  vinit=0.0
  Step : Step  Time=0.000001  Before=1  After=0  SampleTime=0
  IAE : Outport
  MAx : Outport  Port=2
  wires:
  Abs/1 -> Integrator/1
  Abs1/1 -> MinMax Running Resettable/1
  Step/1 -> MinMax Running Resettable/2
  e/1 -> Abs/1, Abs1/1
  Integrator/1 -> IAE/1
  MinMax Running Resettable/1 -> MAx/1

== system Model_4/Subsystem2/Subsystem ==
  ut : Inport
  ul : Inport  Port=2
  Dt : Inport  Port=3
  Add : Sum
  Constant : Constant  Value=-mc*g
  Constant1 : Constant  Value=mc
  Crane : MATLAB Function  TreatAsAtomicUnit=on
  Integrator{,1,3..5} (5 alike) : Integrator
  Integrator2 : Integrator  InitialCondition=l_ini
  x : Outport
  l : Outport  Port=2
  the : Outport  Port=3
  wires:
  Integrator5/1 -> [x6]
  Integrator2/1 -> [x3], l/1
  [x4] -> Crane/3(x4)
  Crane/5(dx5) -> Integrator4/1
  Crane/6(dx6) -> Integrator5/1
  Crane/1(dx1) -> Integrator/1
  Crane/3(dx3) -> Integrator2/1
  Integrator1/1 -> [x2]
  [x2] -> Crane/1(x2)
  Integrator4/1 -> [x5], the/1
  [x3] -> Crane/2(x3)
  [x6] -> Crane/5(x6)
  [x5] -> Crane/4(x5)
  Crane/4(dx4) -> Integrator3/1
  Integrator/1 -> x/1, [x1]
  Integrator3/1 -> [x4]
  Crane/2(dx2) -> Integrator1/1
  ut/1 -> Crane/6(ut)
  ul/1 -> Add/2
  Constant/1 -> Add/1
  Add/1 -> Crane/7(ul)
  Dt/1 -> Crane/8(Dt)
  Constant1/1 -> Crane/9(mc)

== system Model_4/Subsystem3/ADRC  ==
  ref : Inport
  x : Inport  Port=2
  Gain : Gain  Gain=Kp
  Gain1 : Gain  Gain=Kd
  Gain2 : Gain  Gain=1/b0
  Observer : Subsystem
  Sum : Sum  Inputs=|+-
  Sum3 : Sum  Inputs=|+-
  Sum4 : Sum  Inputs=|+-
  u : Outport
  wires:
  Sum4/1 -> Gain2/1
  Sum/1 -> Gain/1
  Gain2/1 -> u/1, Observer/1(u)
  x/1 -> Observer/2(x)
  Sum3/1 -> Sum4/1
  Observer/2(x2) -> Gain1/1
  Gain1/1 -> Sum3/2
  Gain/1 -> Sum3/1
  ref/1 -> Sum/1
  Observer/1(x3) -> Sum4/2
  Observer/3(x1) -> Sum/2

== system Model_4/Subsystem3/ADRC 1 ==
  ref : Inport
  x : Inport  Port=2
  Gain : Gain  Gain=Kp1
  Gain1 : Gain  Gain=Kd1
  Gain2 : Gain  Gain=1/b1
  Observer : Subsystem
  Sum : Sum  Inputs=|+-
  Sum3 : Sum  Inputs=|+-
  Sum4 : Sum  Inputs=|+-
  u : Outport
  wires:
  Sum4/1 -> Gain2/1
  Sum/1 -> Gain/1
  Gain2/1 -> u/1, Observer/1(u)
  x/1 -> Observer/2(x)
  Sum3/1 -> Sum4/1
  Observer/2(x2) -> Gain1/1
  Gain1/1 -> Sum3/2
  Gain/1 -> Sum3/1
  ref/1 -> Sum/1
  Observer/1(x3) -> Sum4/2
  Observer/3(x1) -> Sum/2

== system Model_4/Subsystem3/Fitness APS ZVD ==
  e : Inport
  Abs : Abs
  Abs1 : Abs
  Integrator : Integrator
  MinMax Running Resettable : simulink/Math Operations/MinMax Running Resettable  Function=max  vinit=0.0
  Step : Step  Time=0.000001  Before=1  After=0  SampleTime=0
  IAE : Outport
  MAx : Outport  Port=2
  wires:
  Abs/1 -> Integrator/1
  Abs1/1 -> MinMax Running Resettable/1
  Step/1 -> MinMax Running Resettable/2
  e/1 -> Abs/1, Abs1/1
  Integrator/1 -> IAE/1
  MinMax Running Resettable/1 -> MAx/1

== system Model_4/Subsystem3/Subsystem ==
  Fx : Inport
  Dp : Inport  Port=2
  Fl : Inport  Port=3
  Add : Sum
  Constant : Constant  Value=-mc*g
  Constant1 : Constant  Value=mc
  Crane : MATLAB Function  TreatAsAtomicUnit=on
  Integrator{,1,3..5} (5 alike) : Integrator
  Integrator2 : Integrator  InitialCondition=l_ini
  x : Outport
  l : Outport  Port=2
  the : Outport  Port=3
  wires:
  Integrator5/1 -> [x6]
  Integrator2/1 -> [x3], l/1
  [x4] -> Crane/3(x4)
  Crane/5(dx5) -> Integrator4/1
  Crane/6(dx6) -> Integrator5/1
  Crane/1(dx1) -> Integrator/1
  Crane/3(dx3) -> Integrator2/1
  Integrator1/1 -> [x2]
  [x2] -> Crane/1(x2)
  Integrator4/1 -> the/1, [x5]
  [x3] -> Crane/2(x3)
  [x6] -> Crane/5(x6)
  [x5] -> Crane/4(x5)
  Crane/4(dx4) -> Integrator3/1
  Integrator/1 -> x/1, [x1]
  Integrator3/1 -> [x4]
  Crane/2(dx2) -> Integrator1/1
  Fx/1 -> Crane/6(Fx)
  Dp/1 -> Crane/9(Dp)
  Constant1/1 -> Crane/8(mp)
  Constant/1 -> Add/1
  Fl/1 -> Add/2
  Add/1 -> Crane/7(Fl)

== system Model_4/Subsystem3/ZVD1 ==
  ref : Inport
  Input : Inport  Port=2
  Input1 : Inport  Port=3
  Gain1 : Gain  Gain=0.25
  Gain2 : Gain  Gain=0.5
  Gain3 : Gain  Gain=0.25
  MATLAB Function : MATLAB Function  Commented=on  TreatAsAtomicUnit=on
  MATLAB Function1 : MATLAB Function  Commented=on  TreatAsAtomicUnit=on
  Sum : Sum  Inputs=+++
  Variable Transport Delay : VariableTransportDelay  VariableDelayType=Variable transport delay  MaximumDelay=10
  Variable Transport Delay1 : VariableTransportDelay  VariableDelayType=Variable transport delay  MaximumDelay=10
  ref_AZ : Outport
  wires:
  Gain2/1 -> Variable Transport Delay/1
  Gain1/1 -> Sum/1
  Variable Transport Delay/1 -> Sum/2
  Sum/1 -> ref_AZ/1
  ref/1 -> Gain1/1, Gain3/1, Gain2/1
  Gain3/1 -> Variable Transport Delay1/1
  Variable Transport Delay1/1 -> Sum/3
  Input/1 -> Variable Transport Delay/2
  MATLAB Function1/1(y) -> ?
  Input1/1 -> Variable Transport Delay1/2

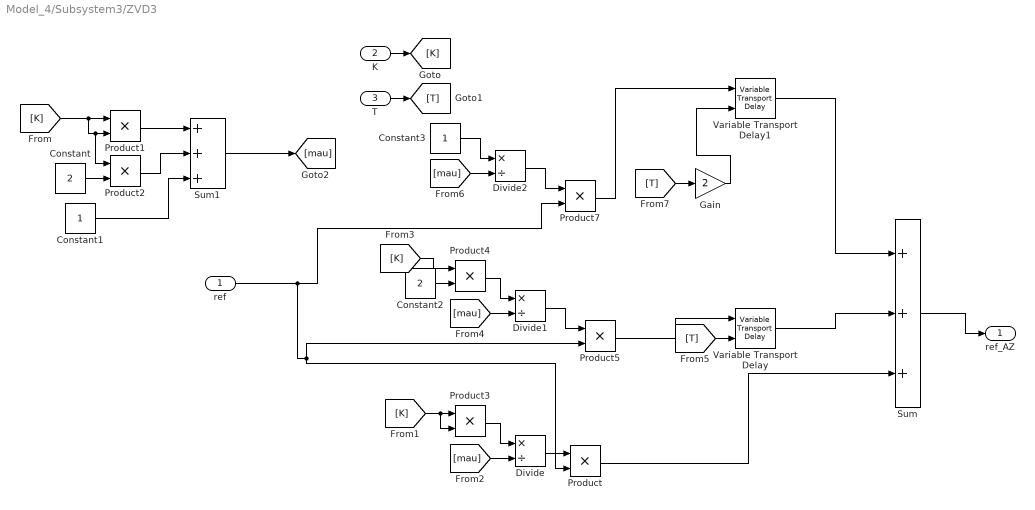
== system Model_4/Subsystem3/ZVD3 ==
  ref : Inport
  K : Inport  Port=2
  T : Inport  Port=3
  Constant : Constant  Value=2
  Constant1 : Constant
  Constant2 : Constant  Value=2
  Constant3 : Constant
  Divide : Product  Inputs=*/
  Divide1 : Product  Inputs=*/
  Divide2 : Product  Inputs=*/
  Gain : Gain  Gain=2
  Product{,1..5,7} (7 alike) : Product
  Sum : Sum  Inputs=+++
  Sum1 : Sum  Inputs=+++
  Variable Transport Delay : VariableTransportDelay  VariableDelayType=Variable transport delay  MaximumDelay=10
  Variable Transport Delay1 : VariableTransportDelay  VariableDelayType=Variable transport delay  MaximumDelay=10
  ref_AZ : Outport
  wires:
  Product5/1 -> Variable Transport Delay/1
  Product7/1 -> Variable Transport Delay1/1
  Variable Transport Delay/1 -> Sum/2
  Sum/1 -> ref_AZ/1
  ref/1 -> Product7/2, Product/2, Product5/2
  Product/1 -> Sum/3
  K/1 -> [K]
  T/1 -> [T]
  [K] -> Product2/1, Product1/2, Product1/1
  Constant/1 -> Product2/2
  Product1/1 -> Sum1/1
  Product2/1 -> Sum1/2
  Constant1/1 -> Sum1/3
  Sum1/1 -> [mau]
  [K] -> Product4/1
  Product4/1 -> Divide1/1
  [mau] -> Divide1/2
  Divide1/1 -> Product5/1
  Constant2/1 -> Product4/2
  Constant3/1 -> Divide2/1
  Divide2/1 -> Product7/1
  [mau] -> Divide2/2
  [K] -> Product3/2, Product3/1
  Product3/1 -> Divide/1
  [mau] -> Divide/2
  Divide/1 -> Product/1
  [T] -> Variable Transport Delay/2
  Gain/1 -> Variable Transport Delay1/2
  [T] -> Gain/1
  Variable Transport Delay1/1 -> Sum/1

== system Model_4/Subsystem3/rbf2_2_5_2 ==
  Input : Inport  PortDimensions=2
      mask Display: e = 0.06;c1 = [120 230 180]/255;c2 = ([120 230 180]+0)/(256+128);c3 = ([120 230 180]+128)/(256+128);patch([0 1 1 0],[0 0 1 1],c1);patch([0 1 1 1-e 1-e 0+e],[0 0 1 1-e 0+e 0+e],c2);patch([0 0 1 1-e 0+e 0+e],[0 1 1 1-e 1-e 0+e],c3);plot([0 1 1 0 0],[0 0 1 1 0]);
  Layer 1 : Subsystem
      mask Display: e = 0.06;c1 = [120 150 230]/255;c2 = ([120 150 230]+0)/383;c3 = ([120 150 230]+128)/383;patch([0 1 1 0],[0 0 1 1],c1);patch([0 1 1 1-e 1-e 0+e],[0 0 1 1-e 0+e 0+e],c2);patch([0 0 1 1-e 0+e 0+e],[0 1 1 1-e 1-e 0+e],c3);plot([0 1 1 0 0],[0 0 1 1 0]);
  Layer 2 : Subsystem
      mask Display: e = 0.06;c1 = [120 150 230]/255;c2 = ([120 150 230]+0)/383;c3 = ([120 150 230]+128)/383;patch([0 1 1 0],[0 0 1 1],c1);patch([0 1 1 1-e 1-e 0+e],[0 0 1 1-e 0+e 0+e],c2);patch([0 0 1 1-e 0+e 0+e],[0 1 1 1-e 1-e 0+e],c3);plot([0 1 1 0 0],[0 0 1 1 0]);
  Process Input 1 : Subsystem
      mask Display: e = 0.06;c1 = [120 150 230]/255;c2 = ([120 150 230]+0)/383;c3 = ([120 150 230]+128)/383;patch([0 1 1 0],[0 0 1 1],c1);patch([0 1 1 1-e 1-e 0+e],[0 0 1 1-e 0+e 0+e],c2);patch([0 0 1 1-e 0+e 0+e],[0 1 1 1-e 1-e 0+e],c3);plot([0 1 1 0 0],[0 0 1 1 0]);
  Process Output 1 : Subsystem
      mask Display: e = 0.06;c1 = [120 150 230]/255;c2 = ([120 150 230]+0)/383;c3 = ([120 150 230]+128)/383;patch([0 1 1 0],[0 0 1 1],c1);patch([0 1 1 1-e 1-e 0+e],[0 0 1 1-e 0+e 0+e],c2);patch([0 0 1 1-e 0+e 0+e],[0 1 1 1-e 1-e 0+e],c3);plot([0 1 1 0 0],[0 0 1 1 0]);
  Output : Outport  InitialOutput=[0;0]
      mask Display: e = 0.06;c1 = [120 230 180]/255;c2 = ([120 230 180]+0)/(256+128);c3 = ([120 230 180]+128)/(256+128);patch([0 1 1 0],[0 0 1 1],c1);patch([0 1 1 1-e 1-e 0+e],[0 0 1 1-e 0+e 0+e],c2);patch([0 0 1 1-e 0+e 0+e],[0 1 1 1-e 1-e 0+e],c3);plot([0 1 1 0 0],[0 0 1 1 0]);
  wires:
  Input/1 -> Process Input 1/1(x)
  Process Output 1/1(y) -> Output/1
  Process Input 1/1(p) -> Layer 1/1("p{1}")
  Layer 1/1("a{1}") -> [feedback1]
  [feedback1] -> Layer 2/1("a{1} ")
  Layer 2/1("a{2}") -> Process Output 1/1(a)

== system Model_4/Subsystem5/ADRC  ==
  ref : Inport
  x : Inport  Port=2
  Gain : Gain  Gain=Kp
  Gain1 : Gain  Gain=Kd
  Gain2 : Gain  Gain=1/b0
  Observer : Subsystem
  Sum : Sum  Inputs=|+-
  Sum3 : Sum  Inputs=|+-
  Sum4 : Sum  Inputs=|+-
  u : Outport
  wires:
  Sum4/1 -> Gain2/1
  Sum/1 -> Gain/1
  Gain2/1 -> u/1, Observer/1(u)
  x/1 -> Observer/2(x)
  Sum3/1 -> Sum4/1
  Observer/2(x2) -> Gain1/1
  Gain1/1 -> Sum3/2
  Gain/1 -> Sum3/1
  ref/1 -> Sum/1
  Observer/1(x3) -> Sum4/2
  Observer/3(x1) -> Sum/2

== system Model_4/Subsystem5/ADRC 1 ==
  ref : Inport
  x : Inport  Port=2
  Gain : Gain  Gain=Kp1
  Gain1 : Gain  Gain=Kd1
  Gain2 : Gain  Gain=1/b1
  Observer : Subsystem
  Sum : Sum  Inputs=|+-
  Sum3 : Sum  Inputs=|+-
  Sum4 : Sum  Inputs=|+-
  u : Outport
  wires:
  Sum4/1 -> Gain2/1
  Sum/1 -> Gain/1
  Gain2/1 -> u/1, Observer/1(u)
  x/1 -> Observer/2(x)
  Sum3/1 -> Sum4/1
  Observer/2(x2) -> Gain1/1
  Gain1/1 -> Sum3/2
  Gain/1 -> Sum3/1
  ref/1 -> Sum/1
  Observer/1(x3) -> Sum4/2
  Observer/3(x1) -> Sum/2

== system Model_4/Subsystem5/Fitness APS ZVD ==
  e : Inport
  Abs : Abs
  Abs1 : Abs
  Integrator : Integrator
  MinMax Running Resettable : simulink/Math Operations/MinMax Running Resettable  Function=max  vinit=0.0
  Step : Step  Time=0.000001  Before=1  After=0  SampleTime=0
  IAE : Outport
  MAx : Outport  Port=2
  wires:
  Abs/1 -> Integrator/1
  Abs1/1 -> MinMax Running Resettable/1
  Step/1 -> MinMax Running Resettable/2
  e/1 -> Abs/1, Abs1/1
  Integrator/1 -> IAE/1
  MinMax Running Resettable/1 -> MAx/1

== system Model_4/Subsystem5/Radial Basis Network ==
  Input : Inport  PortDimensions=2
      mask Display: e = 0.06;c1 = [120 230 180]/255;c2 = ([120 230 180]+0)/(256+128);c3 = ([120 230 180]+128)/(256+128);patch([0 1 1 0],[0 0 1 1],c1);patch([0 1 1 1-e 1-e 0+e],[0 0 1 1-e 0+e 0+e],c2);patch([0 0 1 1-e 0+e 0+e],[0 1 1 1-e 1-e 0+e],c3);plot([0 1 1 0 0],[0 0 1 1 0]);
  Layer 1 : Subsystem
      mask Display: e = 0.06;c1 = [120 150 230]/255;c2 = ([120 150 230]+0)/383;c3 = ([120 150 230]+128)/383;patch([0 1 1 0],[0 0 1 1],c1);patch([0 1 1 1-e 1-e 0+e],[0 0 1 1-e 0+e 0+e],c2);patch([0 0 1 1-e 0+e 0+e],[0 1 1 1-e 1-e 0+e],c3);plot([0 1 1 0 0],[0 0 1 1 0]);
  Layer 2 : Subsystem
      mask Display: e = 0.06;c1 = [120 150 230]/255;c2 = ([120 150 230]+0)/383;c3 = ([120 150 230]+128)/383;patch([0 1 1 0],[0 0 1 1],c1);patch([0 1 1 1-e 1-e 0+e],[0 0 1 1-e 0+e 0+e],c2);patch([0 0 1 1-e 0+e 0+e],[0 1 1 1-e 1-e 0+e],c3);plot([0 1 1 0 0],[0 0 1 1 0]);
  Process Input 1 : Subsystem
      mask Display: e = 0.06;c1 = [120 150 230]/255;c2 = ([120 150 230]+0)/383;c3 = ([120 150 230]+128)/383;patch([0 1 1 0],[0 0 1 1],c1);patch([0 1 1 1-e 1-e 0+e],[0 0 1 1-e 0+e 0+e],c2);patch([0 0 1 1-e 0+e 0+e],[0 1 1 1-e 1-e 0+e],c3);plot([0 1 1 0 0],[0 0 1 1 0]);
  Process Output 1 : Subsystem
      mask Display: e = 0.06;c1 = [120 150 230]/255;c2 = ([120 150 230]+0)/383;c3 = ([120 150 230]+128)/383;patch([0 1 1 0],[0 0 1 1],c1);patch([0 1 1 1-e 1-e 0+e],[0 0 1 1-e 0+e 0+e],c2);patch([0 0 1 1-e 0+e 0+e],[0 1 1 1-e 1-e 0+e],c3);plot([0 1 1 0 0],[0 0 1 1 0]);
  Output : Outport  InitialOutput=[0;0]
      mask Display: e = 0.06;c1 = [120 230 180]/255;c2 = ([120 230 180]+0)/(256+128);c3 = ([120 230 180]+128)/(256+128);patch([0 1 1 0],[0 0 1 1],c1);patch([0 1 1 1-e 1-e 0+e],[0 0 1 1-e 0+e 0+e],c2);patch([0 0 1 1-e 0+e 0+e],[0 1 1 1-e 1-e 0+e],c3);plot([0 1 1 0 0],[0 0 1 1 0]);
  wires:
  Input/1 -> Process Input 1/1(x)
  Process Output 1/1(y) -> Output/1
  Process Input 1/1(p) -> Layer 1/1("p{1}")
  Layer 1/1("a{1}") -> [feedback1]
  [feedback1] -> Layer 2/1("a{1} ")
  Layer 2/1("a{2}") -> Process Output 1/1(a)

== system Model_4/Subsystem5/Subsystem ==
  Fx : Inport
  Fl : Inport  Port=2
  Dp : Inport  Port=3
  Add : Sum
  Constant : Constant  Value=-mc*g
  Constant1 : Constant  Value=mc
  Crane : MATLAB Function  TreatAsAtomicUnit=on
  Integrator{,1,3..5} (5 alike) : Integrator
  Integrator2 : Integrator  InitialCondition=l_ini
  Scope : Scope
  x : Outport
  l : Outport  Port=2
  the : Outport  Port=3
  wires:
  Integrator5/1 -> [x6]
  Integrator2/1 -> l/1, [x3]
  [x4] -> Crane/3(x4)
  Crane/5(dx5) -> Integrator4/1
  Crane/6(dx6) -> Integrator5/1
  Crane/1(dx1) -> Scope/1, Integrator/1
  Crane/3(dx3) -> Integrator2/1
  Integrator1/1 -> [x2]
  [x2] -> Crane/1(x2)
  Integrator4/1 -> the/1, [x5]
  [x3] -> Crane/2(x3)
  [x6] -> Crane/5(x6)
  [x5] -> Crane/4(x5)
  Crane/4(dx4) -> Integrator3/1
  Integrator/1 -> x/1, [x1]
  Integrator3/1 -> [x4]
  Crane/2(dx2) -> Integrator1/1
  Fx/1 -> Crane/6(Fx)
  Fl/1 -> Add/2
  Constant/1 -> Add/1
  Add/1 -> Crane/7(Fl)
  Dp/1 -> Crane/8(Dp)
  Constant1/1 -> Crane/9(mp)

== system Model_4/Subsystem5/ZVD1 ==
  ref : Inport
  Input : Inport  Port=2
  Input1 : Inport  Port=3
  Gain1 : Gain  Gain=0.25
  Gain2 : Gain  Gain=0.5
  Gain3 : Gain  Gain=0.25
  MATLAB Function : MATLAB Function  Commented=on  TreatAsAtomicUnit=on
  MATLAB Function1 : MATLAB Function  Commented=on  TreatAsAtomicUnit=on
  Sum : Sum  Inputs=+++
  Variable Transport Delay : VariableTransportDelay  VariableDelayType=Variable transport delay  MaximumDelay=10
  Variable Transport Delay1 : VariableTransportDelay  VariableDelayType=Variable transport delay  MaximumDelay=10
  ref_AZ : Outport
  wires:
  Gain2/1 -> Variable Transport Delay/1
  Gain1/1 -> Sum/1
  Variable Transport Delay/1 -> Sum/2
  Sum/1 -> ref_AZ/1
  ref/1 -> Gain1/1, Gain3/1, Gain2/1
  Gain3/1 -> Variable Transport Delay1/1
  Variable Transport Delay1/1 -> Sum/3
  Input/1 -> Variable Transport Delay/2
  MATLAB Function1/1(y) -> ?
  Input1/1 -> Variable Transport Delay1/2

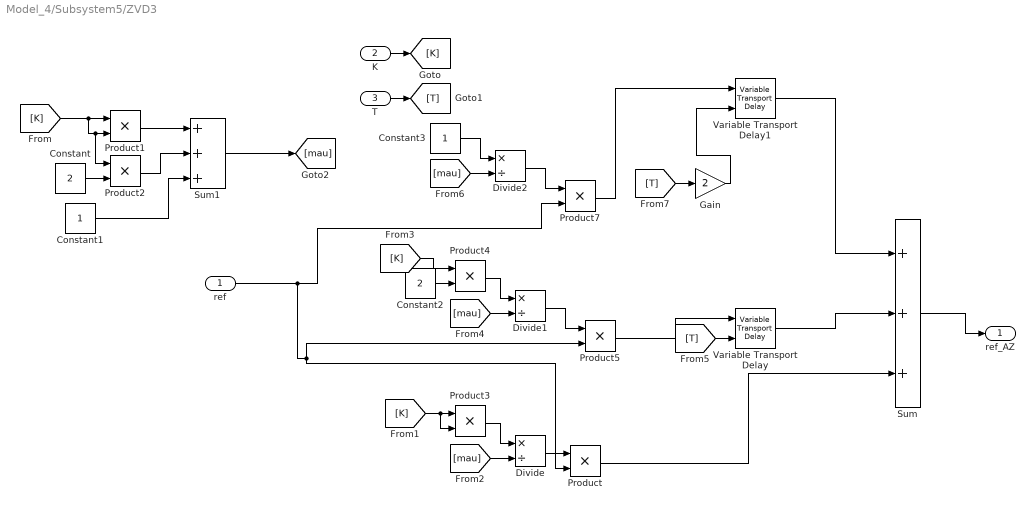
== system Model_4/Subsystem5/ZVD3 ==
  ref : Inport
  K : Inport  Port=2
  T : Inport  Port=3
  Constant : Constant  Value=2
  Constant1 : Constant
  Constant2 : Constant  Value=2
  Constant3 : Constant
  Divide : Product  Inputs=*/
  Divide1 : Product  Inputs=*/
  Divide2 : Product  Inputs=*/
  Gain : Gain  Gain=2
  Product{,1..5,7} (7 alike) : Product
  Sum : Sum  Inputs=+++
  Sum1 : Sum  Inputs=+++
  Variable Transport Delay : VariableTransportDelay  VariableDelayType=Variable transport delay  MaximumDelay=10
  Variable Transport Delay1 : VariableTransportDelay  VariableDelayType=Variable transport delay  MaximumDelay=10
  ref_AZ : Outport
  wires:
  Product5/1 -> Variable Transport Delay/1
  Product7/1 -> Variable Transport Delay1/1
  Variable Transport Delay/1 -> Sum/2
  Sum/1 -> ref_AZ/1
  ref/1 -> Product7/2, Product/2, Product5/2
  Product/1 -> Sum/3
  K/1 -> [K]
  T/1 -> [T]
  [K] -> Product2/1, Product1/2, Product1/1
  Constant/1 -> Product2/2
  Product1/1 -> Sum1/1
  Product2/1 -> Sum1/2
  Constant1/1 -> Sum1/3
  Sum1/1 -> [mau]
  [K] -> Product4/1
  Product4/1 -> Divide1/1
  [mau] -> Divide1/2
  Divide1/1 -> Product5/1
  Constant2/1 -> Product4/2
  Constant3/1 -> Divide2/1
  Divide2/1 -> Product7/1
  [mau] -> Divide2/2
  [K] -> Product3/2, Product3/1
  Product3/1 -> Divide/1
  [mau] -> Divide/2
  Divide/1 -> Product/1
  [T] -> Variable Transport Delay/2
  Gain/1 -> Variable Transport Delay1/2
  [T] -> Gain/1
  Variable Transport Delay1/1 -> Sum/1

== system Model_4/AOF/ADRC 1/Observer ==
  u : Inport
  x : Inport  Port=2
  Gain : Gain  Gain=-l11
  Gain1 : Gain  Gain=l11
  Gain2 : Gain  Gain=-l21
  Gain3 : Gain  Gain=l21
  Gain4 : Gain  Gain=-l31
  Gain5 : Gain  Gain=l31
  Gain6 : Gain  Gain=b1
  Integrator : Integrator  InitialCondition=l_ini
  Integrator1 : Integrator
  Integrator2 : Integrator
  Sum : Sum  Inputs=+++
  Sum1 : Sum  Inputs=++++
  Sum2 : Sum
  x3 : Outport
  x2 : Outport  Port=2
  x1 : Outport  Port=3
  wires:
  Sum2/1 -> Integrator2/1
  [x21] -> Sum/2
  Integrator2/1 -> [x31], x3/1
  x/1 -> Gain1/1, Gain5/1, Gain3/1
  Gain1/1 -> Sum/3
  Sum/1 -> Integrator/1
  Gain4/1 -> Sum2/1
  [x11] -> Gain4/1
  Gain5/1 -> Sum2/2
  Integrator1/1 -> [x21], x2/1
  Gain6/1 -> Sum1/3
  Gain/1 -> Sum/1
  Integrator/1 -> [x11], x1/1
  [x31] -> Sum1/2
  u/1 -> Gain6/1
  Gain2/1 -> Sum1/1
  Sum1/1 -> Integrator1/1
  [x11] -> Gain2/1
  [x11] -> Gain/1
  Gain3/1 -> Sum1/4

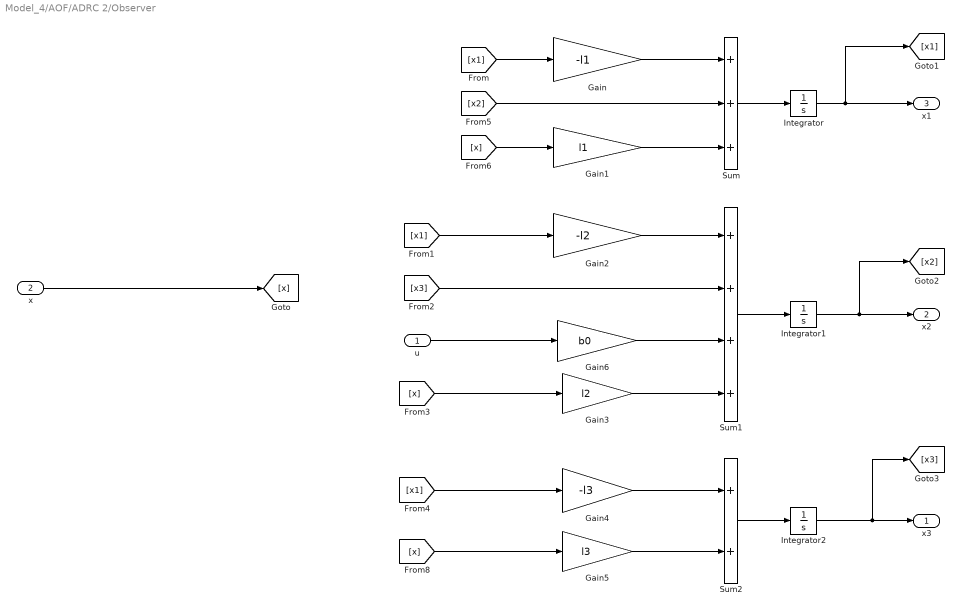
== system Model_4/AOF/ADRC 2/Observer ==
  u : Inport
  x : Inport  Port=2
  Gain : Gain  Gain=-l1
  Gain1 : Gain  Gain=l1
  Gain2 : Gain  Gain=-l2
  Gain3 : Gain  Gain=l2
  Gain4 : Gain  Gain=-l3
  Gain5 : Gain  Gain=l3
  Gain6 : Gain  Gain=b0
  Integrator : Integrator
  Integrator1 : Integrator
  Integrator2 : Integrator
  Sum : Sum  Inputs=+++
  Sum1 : Sum  Inputs=++++
  Sum2 : Sum
  x3 : Outport
  x2 : Outport  Port=2
  x1 : Outport  Port=3
  wires:
  Sum2/1 -> Integrator2/1
  [x2] -> Sum/2
  Integrator2/1 -> [x3], x3/1
  [x] -> Gain5/1
  [x] -> Gain1/1
  Gain1/1 -> Sum/3
  Sum/1 -> Integrator/1
  Gain4/1 -> Sum2/1
  [x1] -> Gain4/1
  Gain5/1 -> Sum2/2
  Integrator1/1 -> [x2], x2/1
  Gain6/1 -> Sum1/3
  Gain/1 -> Sum/1
  Integrator/1 -> [x1], x1/1
  [x3] -> Sum1/2
  [x] -> Gain3/1
  u/1 -> Gain6/1
  Gain2/1 -> Sum1/1
  Sum1/1 -> Integrator1/1
  [x1] -> Gain2/1
  [x1] -> Gain/1
  x/1 -> [x]
  Gain3/1 -> Sum1/4

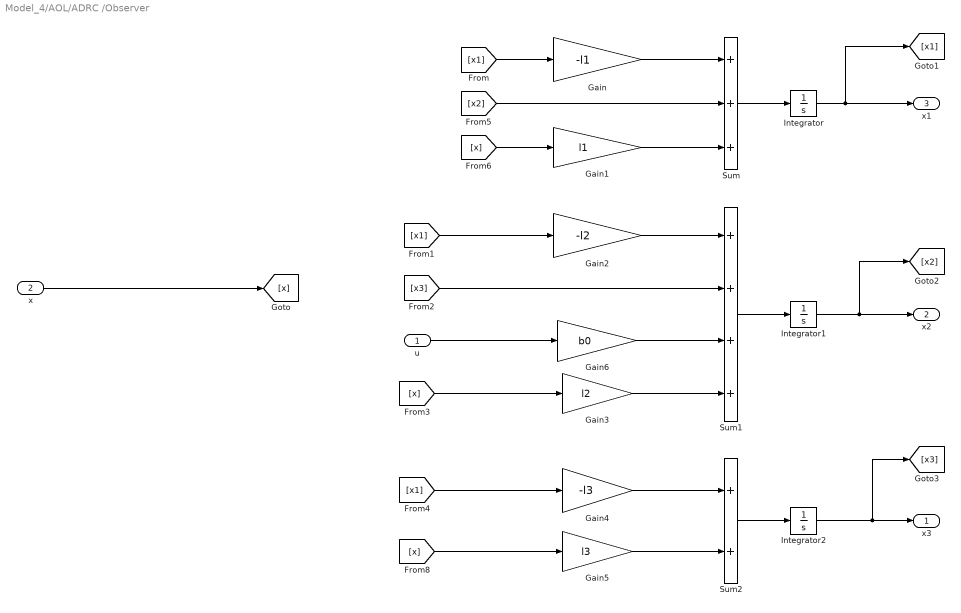
== system Model_4/AOL/ADRC /Observer ==
  u : Inport
  x : Inport  Port=2
  Gain : Gain  Gain=-l1
  Gain1 : Gain  Gain=l1
  Gain2 : Gain  Gain=-l2
  Gain3 : Gain  Gain=l2
  Gain4 : Gain  Gain=-l3
  Gain5 : Gain  Gain=l3
  Gain6 : Gain  Gain=b0
  Integrator : Integrator
  Integrator1 : Integrator
  Integrator2 : Integrator
  Sum : Sum  Inputs=+++
  Sum1 : Sum  Inputs=++++
  Sum2 : Sum
  x3 : Outport
  x2 : Outport  Port=2
  x1 : Outport  Port=3
  wires:
  Sum2/1 -> Integrator2/1
  [x2] -> Sum/2
  Integrator2/1 -> [x3], x3/1
  [x] -> Gain5/1
  [x] -> Gain1/1
  Gain1/1 -> Sum/3
  Sum/1 -> Integrator/1
  Gain4/1 -> Sum2/1
  [x1] -> Gain4/1
  Gain5/1 -> Sum2/2
  Integrator1/1 -> [x2], x2/1
  Gain6/1 -> Sum1/3
  Gain/1 -> Sum/1
  Integrator/1 -> [x1], x1/1
  [x3] -> Sum1/2
  [x] -> Gain3/1
  u/1 -> Gain6/1
  Gain2/1 -> Sum1/1
  Sum1/1 -> Integrator1/1
  [x1] -> Gain2/1
  [x1] -> Gain/1
  x/1 -> [x]
  Gain3/1 -> Sum1/4

== system Model_4/AOL/ADRC 1/Observer ==
  u : Inport
  x : Inport  Port=2
  Gain : Gain  Gain=-l11
  Gain1 : Gain  Gain=l11
  Gain2 : Gain  Gain=-l21
  Gain3 : Gain  Gain=l21
  Gain4 : Gain  Gain=-l31
  Gain5 : Gain  Gain=l31
  Gain6 : Gain  Gain=b1
  Integrator : Integrator  InitialCondition=l_ini
  Integrator1 : Integrator
  Integrator2 : Integrator
  Sum : Sum  Inputs=+++
  Sum1 : Sum  Inputs=++++
  Sum2 : Sum
  x3 : Outport
  x2 : Outport  Port=2
  x1 : Outport  Port=3
  wires:
  Sum2/1 -> Integrator2/1
  [x21] -> Sum/2
  Integrator2/1 -> [x31], x3/1
  x/1 -> Gain1/1, Gain5/1, Gain3/1
  Gain1/1 -> Sum/3
  Sum/1 -> Integrator/1
  Gain4/1 -> Sum2/1
  [x11] -> Gain4/1
  Gain5/1 -> Sum2/2
  Integrator1/1 -> [x21], x2/1
  Gain6/1 -> Sum1/3
  Gain/1 -> Sum/1
  Integrator/1 -> [x11], x1/1
  [x31] -> Sum1/2
  u/1 -> Gain6/1
  Gain2/1 -> Sum1/1
  Sum1/1 -> Integrator1/1
  [x11] -> Gain2/1
  [x11] -> Gain/1
  Gain3/1 -> Sum1/4

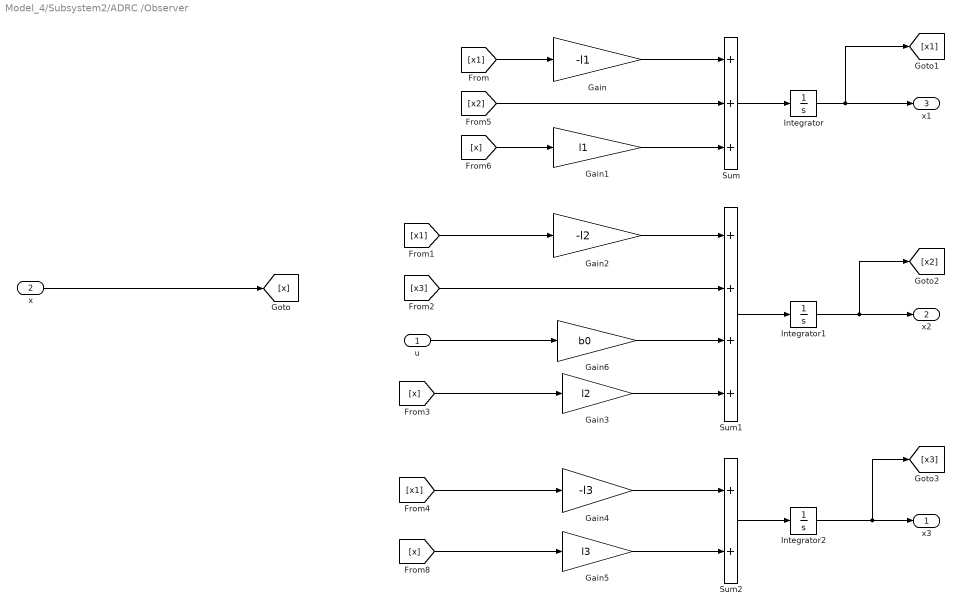
== system Model_4/Subsystem2/ADRC /Observer ==
  u : Inport
  x : Inport  Port=2
  Gain : Gain  Gain=-l1
  Gain1 : Gain  Gain=l1
  Gain2 : Gain  Gain=-l2
  Gain3 : Gain  Gain=l2
  Gain4 : Gain  Gain=-l3
  Gain5 : Gain  Gain=l3
  Gain6 : Gain  Gain=b0
  Integrator : Integrator
  Integrator1 : Integrator
  Integrator2 : Integrator
  Sum : Sum  Inputs=+++
  Sum1 : Sum  Inputs=++++
  Sum2 : Sum
  x3 : Outport
  x2 : Outport  Port=2
  x1 : Outport  Port=3
  wires:
  Sum2/1 -> Integrator2/1
  [x2] -> Sum/2
  Integrator2/1 -> [x3], x3/1
  [x] -> Gain5/1
  [x] -> Gain1/1
  Gain1/1 -> Sum/3
  Sum/1 -> Integrator/1
  Gain4/1 -> Sum2/1
  [x1] -> Gain4/1
  Gain5/1 -> Sum2/2
  Integrator1/1 -> [x2], x2/1
  Gain6/1 -> Sum1/3
  Gain/1 -> Sum/1
  Integrator/1 -> [x1], x1/1
  [x3] -> Sum1/2
  [x] -> Gain3/1
  u/1 -> Gain6/1
  Gain2/1 -> Sum1/1
  Sum1/1 -> Integrator1/1
  [x1] -> Gain2/1
  [x1] -> Gain/1
  x/1 -> [x]
  Gain3/1 -> Sum1/4

== system Model_4/Subsystem2/ADRC 1/Observer ==
  u : Inport
  x : Inport  Port=2
  Gain : Gain  Gain=-l11
  Gain1 : Gain  Gain=l11
  Gain2 : Gain  Gain=-l21
  Gain3 : Gain  Gain=l21
  Gain4 : Gain  Gain=-l31
  Gain5 : Gain  Gain=l31
  Gain6 : Gain  Gain=b1
  Integrator : Integrator  InitialCondition=l_ini
  Integrator1 : Integrator
  Integrator2 : Integrator
  Sum : Sum  Inputs=+++
  Sum1 : Sum  Inputs=++++
  Sum2 : Sum
  x3 : Outport
  x2 : Outport  Port=2
  x1 : Outport  Port=3
  wires:
  Sum2/1 -> Integrator2/1
  [x21] -> Sum/2
  Integrator2/1 -> [x31], x3/1
  x/1 -> Gain1/1, Gain5/1, Gain3/1
  Gain1/1 -> Sum/3
  Sum/1 -> Integrator/1
  Gain4/1 -> Sum2/1
  [x11] -> Gain4/1
  Gain5/1 -> Sum2/2
  Integrator1/1 -> [x21], x2/1
  Gain6/1 -> Sum1/3
  Gain/1 -> Sum/1
  Integrator/1 -> [x11], x1/1
  [x31] -> Sum1/2
  u/1 -> Gain6/1
  Gain2/1 -> Sum1/1
  Sum1/1 -> Integrator1/1
  [x11] -> Gain2/1
  [x11] -> Gain/1
  Gain3/1 -> Sum1/4
